simulink model "simlab6d"  (R2021a)
settings: Solver=ode4  StartTime=0.0  StopTime=10.0  FixedStep=0.001  RelTol=1e-3
values from neighbouring files (symbols this model uses):
  B = Bm+KT*KB/Ra+N^2*BL    (= 0.00447530013037)    [cslab8.m]
  J = Jm+N^2*JL    (= 0.000197449330572)    [cslab8.m]
  K = KT/Ra    (= 0.0210465116279)    [cslab8.m]
  K1 = wn^2*J/(Kp*K)    [cslab8.m]
  Kd = K2*KTG/Kp    [cslab8.m]
  Kp = 0.36    [cslab8.m]
settings Model: Creator=martinsundar  LastModifiedBy=martinsundar

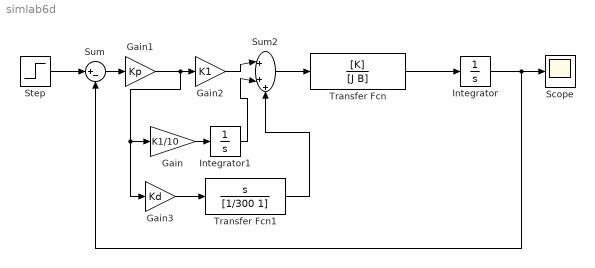
== system simlab6d ==
  Gain : Gain  Gain=K1/10
  Gain1 : Gain  Gain=Kp
  Gain2 : Gain  Gain=K1
  Gain3 : Gain  Gain=Kd
  Integrator : Integrator
  Integrator1 : Integrator
  Scope : Scope
  Step : Step  Time=0  SampleTime=0
  Sum : Sum  Inputs=|+-
  Sum2 : Sum  Inputs=|+++
  Transfer Fcn : TransferFcn  Numerator=[K]  Denominator=[J B]
  Transfer Fcn1 : TransferFcn  Numerator=[1 0]  Denominator=[1/300 1]
  wires:
  Step/1 -> Sum/1
  Sum2/1 -> Transfer Fcn/1
  Transfer Fcn/1 -> Integrator/1
  Integrator/1 -> Sum/2, Scope/1
  Sum/1 -> Gain1/1
  Gain/1 -> Integrator1/1
  Integrator1/1 -> Sum2/2
  Gain2/1 -> Sum2/1
  Gain1/1 -> Gain3/1, Gain/1, Gain2/1
  Transfer Fcn1/1 -> Sum2/3
  Gain3/1 -> Transfer Fcn1/1
